simulink model "microgrid_ex"  (R2020a)
settings: Solver=VariableStepAuto  StartTime=0.0  StopTime=10.0  RelTol=1e-3
libraries: exampleMicrogridLibrary x10, powerlib x4
settings Model: Creator=ramaz  LastModifiedBy=ramaz

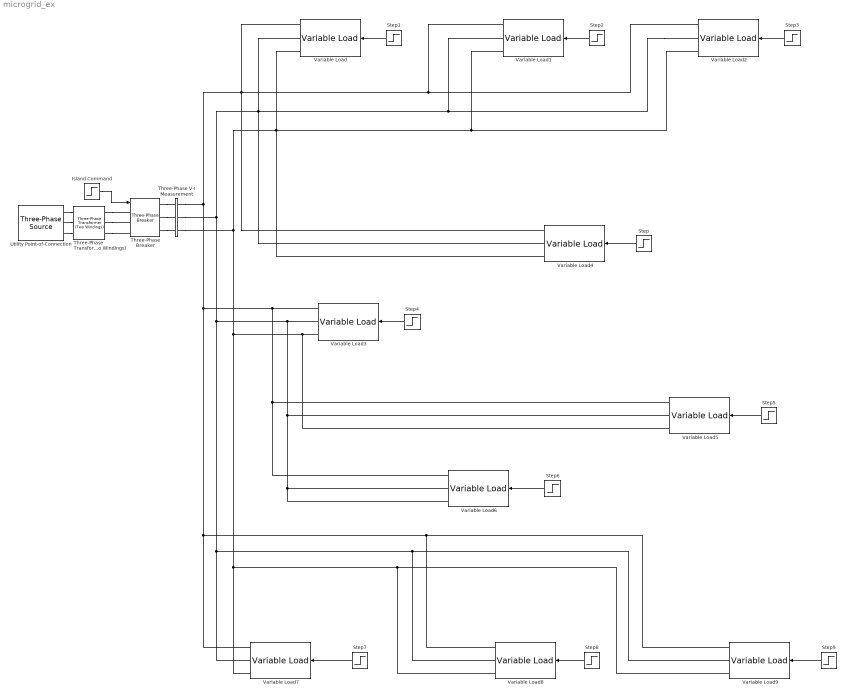
== system microgrid_ex ==
  Island Command : Step  Time=15  Before=1  After=0  SampleTime=0
  Step{,1..9} (10 alike) : Step  SampleTime=0
  Three-Phase Transformer (Two Windings) : powerlib/Elements/Three-Phase Transformer (Two Windings)  Winding1Connection=Yg  Winding2Connection=Yg  CoreType=Three single-phase transformers  SetSaturation=off  Hysteresis=off  DataFile='hysteresis'  SetInitialFlux=off  Measurements=None  UNITS=pu  NominalPower=[ 250e6 , 60 ]  Winding1=[ 13.8e3 , 0.002 , 0.08 ]  Winding2=[ 5000 , 0.002 , 0.08 ]  Rm=500  Lm=500  L0=0.5  Saturation=[ 0,0 ; 0.0024,1.2 ; 1.0,1.52 ]  InitialFluxes=[ 0.8 , -0.8 , 0.7 ]  BreakLoop=off  DiscreteSolver=Trapezoidal iterative  DataType=off  TransfoNumber=1
  Three-Phase V-I Measurement : powerlib/Measurements/Three-Phase V-I Measurement  VoltageMeasurement=phase-to-ground  SetLabelV=on  LabelV=Vabc  Vpu=off  VpuLL=off  CurrentMeasurement=yes  SetLabelI=on  LabelI=Iabc  Ipu=off  Pbase=100e6  Vbase=500e3  OutputType=Complex  PhasorSimulation=off  PSBequivalent=0
  Three-Phase Breaker : powerlib/Elements/Three-Phase Breaker  InitialState=closed  SwitchA=on  SwitchB=on  SwitchC=on  SwitchTimes="[1/60  5/60]"  External=on  BreakerResistance=0.01  SnubberResistance=1e6  SnubberCapacitance=inf  Measurements=None
  Utility Point-of-Connection : powerlib/Electrical Sources/Three-Phase Source  InternalConnection=Yg  VoltagePhases=off  Voltage=(13800)*1.00243  PhaseAngle=0.071468  Voltage_phases=[25e3 25e3 25e3]/sqrt(3)  PhaseAngles_phases=[0 -120 +120]  Frequency=60  NonIdealSource=on  SpecifyImpedance=on  Resistance=0.8929  Inductance=16.58e-3  ShortCircuitLevel=250e6  BaseVoltage=13.8e3  XRratio=7  BusType=swing  Pref=10e3  Qref=0  Prefabc=[10e3, 10e3, 10e3]  Qrefabc=[0, 0, 0]  Qmin=-inf  Qmax=inf
  Variable Load{,1..9} (10 alike) : exampleMicrogridLibrary/Variable Load  Vn=5000  Fn=60  PF=1  Load0=200e3
  wires:
  Island Command/1 -> Three-Phase Breaker/1
  Step1/1 -> Variable Load/1
  Step2/1 -> Variable Load1/1
  Step3/1 -> Variable Load2/1
  Step/1 -> Variable Load4/1
  Step4/1 -> Variable Load3/1
  Step5/1 -> Variable Load5/1
  Step6/1 -> Variable Load6/1
  Step7/1 -> Variable Load7/1
  Step8/1 -> Variable Load8/1
  Step9/1 -> Variable Load9/1
  connections:
  Three-Phase Breaker/RConn2 -- Three-Phase V-I Measurement/LConn2
  Three-Phase Transformer (Two Windings)/RConn3 -- Three-Phase Breaker/LConn3
  Three-Phase Transformer (Two Windings)/RConn2 -- Three-Phase Breaker/LConn2
  Three-Phase Transformer (Two Windings)/RConn1 -- Three-Phase Breaker/LConn1
  Utility Point-of-Connection/RConn3 -- Three-Phase Transformer (Two Windings)/LConn3
  Utility Point-of-Connection/RConn2 -- Three-Phase Transformer (Two Windings)/LConn2
  Utility Point-of-Connection/RConn1 -- Three-Phase Transformer (Two Windings)/LConn1
  Three-Phase Breaker/RConn1 -- Three-Phase V-I Measurement/LConn1
  Three-Phase Breaker/RConn3 -- Three-Phase V-I Measurement/LConn3
  Three-Phase V-I Measurement/RConn1 -- Variable Load8/RConn1 -- Variable Load9/RConn1 -- Variable Load7/RConn1 -- Variable Load6/RConn1 -- Variable Load5/RConn1 -- Variable Load3/RConn1 -- Variable Load2/RConn1 -- Variable Load1/RConn1 -- Variable Load/RConn1 -- Variable Load4/RConn1
  Three-Phase V-I Measurement/RConn2 -- Variable Load8/RConn2 -- Variable Load9/RConn2 -- Variable Load7/RConn2 -- Variable Load6/RConn3 -- Variable Load6/RConn2 -- Variable Load5/RConn2 -- Variable Load3/RConn2 -- Variable Load2/RConn2 -- Variable Load1/RConn2 -- Variable Load/RConn2 -- Variable Load4/RConn2
  Three-Phase V-I Measurement/RConn3 -- Variable Load9/RConn3 -- Variable Load8/RConn3 -- Variable Load7/RConn3 -- Variable Load5/RConn3 -- Variable Load3/RConn3 -- Variable Load2/RConn3 -- Variable Load1/RConn3 -- Variable Load/RConn3 -- Variable Load4/RConn3
